simulink model "OPSPACE_Control"  (R2022b)
settings: Solver=VariableStepAuto  StartTime=0.0  StopTime=70  RelTol=1e-3
values from neighbouring files (symbols this model uses):
  a1 = 0.5    [MODELLO_ROBOT.m]    (also in calcoloJa.m)
  a2 = 0.5    [MODELLO_ROBOT.m]    (also in calcoloJa.m)
  d0 = 1    [MODELLO_ROBOT.m]    (also in calcoloJa.m)
  Kd = diag([50 50 50 50])    [MAIN.m]
  Kp = diag([750 750 750 750])    [MAIN.m]
  q0 = [theta10; theta20; p0(3)-1; -theta10-theta20]    [MAIN.m]
undefined symbols (not defined in the file or in its folder): DiscIntNeverNeededParam
settings Model: Creator=salvatoregranata  LastModifiedBy=salvatoregranata

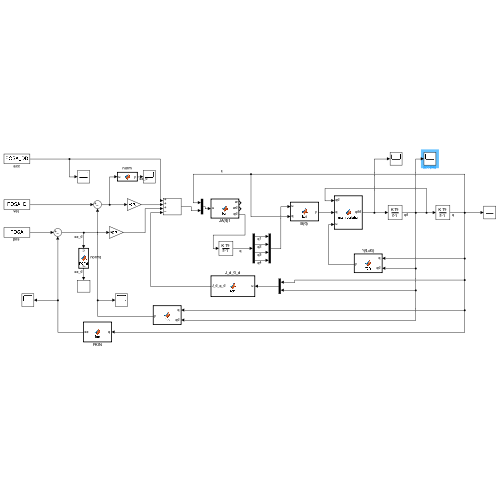
[thumbnail: Simulink's stored preview of the top-level diagram]
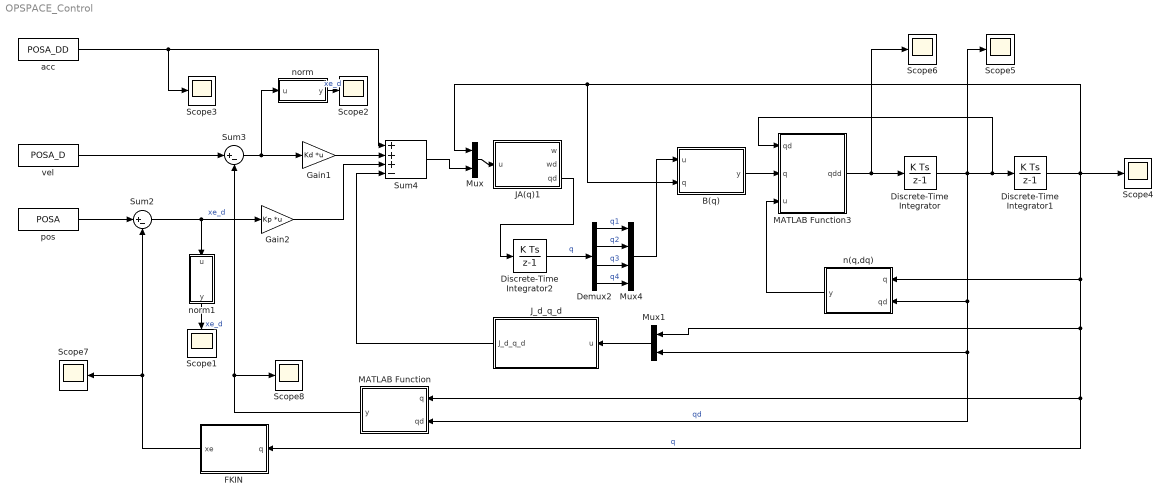
== system OPSPACE_Control ==
  B(q) : MATLAB Function  TreatAsAtomicUnit=on
  Demux2 : Demux
  Discrete-Time Integrator : DiscreteIntegrator  InitialCondition=zeros(1,4)  SampleTime=1e-3  ICPrevOutput=DiscIntNeverNeededParam  ICPrevScaledInput=DiscIntNeverNeededParam
  Discrete-Time Integrator1 : DiscreteIntegrator  InitialCondition=zeros(1,4)  SampleTime=1e-3  ICPrevOutput=DiscIntNeverNeededParam  ICPrevScaledInput=DiscIntNeverNeededParam
  Discrete-Time Integrator2 : DiscreteIntegrator  InitialCondition=q0  SampleTime=1e-3  ICPrevOutput=DiscIntNeverNeededParam  ICPrevScaledInput=DiscIntNeverNeededParam
  FKIN : MATLAB Function  TreatAsAtomicUnit=on
  Gain1 : Gain  Gain=Kd  Multiplication=Matrix(K*u)
  Gain2 : Gain  Gain=Kp  Multiplication=Matrix(K*u)
  JA(q)1 : MATLAB Function  TreatAsAtomicUnit=on
  J_d_q_d : MATLAB Function  TreatAsAtomicUnit=on
  MATLAB Function : MATLAB Function  TreatAsAtomicUnit=on
  MATLAB Function3 : MATLAB Function  TreatAsAtomicUnit=on
  Mux : Mux  Inputs=2
  Mux1 : Mux  Inputs=2
  Mux4 : Mux
  Scope{1..8} (8 alike) : Scope
  Sum2 : Sum  Inputs=|+-
  Sum3 : Sum  Inputs=|+-
  Sum4 : Sum  Inputs=+++-
  acc : FromWorkspace  VariableName=POSA_DD  SampleTime=0.001
  n(q,dq) : MATLAB Function  TreatAsAtomicUnit=on
  norm : MATLAB Function  TreatAsAtomicUnit=on
  norm1 : MATLAB Function  TreatAsAtomicUnit=on
  "pos " : FromWorkspace  VariableName=POSA  SampleTime=0.001
  "vel " : FromWorkspace  VariableName=POSA_D  SampleTime=0.001
  wires:
  acc/1 -> Scope3/1, Sum4/1
  Gain2/1 -> Sum4/3
  "pos "/1 -> Sum2/1
  Gain1/1 -> Sum4/2
  Sum3/1 -> Gain1/1, norm/1(u)
  "vel "/1 -> Sum3/1
  J_d_q_d/1(J_d_q_d) -> Sum4/4
  FKIN/1(xe) -> Scope7/1, Sum2/2
  B(q)/1(y) -> MATLAB Function3/2(q)
  MATLAB Function3/1(qdd) -> Scope6/1, Discrete-Time Integrator/1
  Discrete-Time Integrator/1 -> MATLAB Function/2(qd), Mux1/2, n(q,dq)/2(qd), Scope5/1, MATLAB Function3/1(qd), Discrete-Time Integrator1/1  "qd"
  n(q,dq)/1(y) -> MATLAB Function3/3(u)
  Discrete-Time Integrator1/1 -> Mux/1, B(q)/2(q), Scope4/1, Mux1/1, MATLAB Function/1(q), FKIN/1(q), n(q,dq)/1(q)  "q"
  MATLAB Function/1(y) -> Scope8/1, Sum3/2
  Mux/1 -> JA(q)1/1(u)
  Sum4/1 -> Mux/2
  Mux1/1 -> J_d_q_d/1(u)
  JA(q)1/3(qd) -> Discrete-Time Integrator2/1
  Demux2/1 -> Mux4/1  "q1"
  Demux2/3 -> Mux4/3  "q3"
  Demux2/4 -> Mux4/4  "q4"
  Discrete-Time Integrator2/1 -> Demux2/1  "q"
  Demux2/2 -> Mux4/2  "q2"
  Mux4/1 -> B(q)/1(u)
  norm/1(y) -> Scope2/1  "xe_d"
  Sum2/1 -> norm1/1(u), Gain2/1  "xe_d"
  norm1/1(y) -> Scope1/1  "xe_d"

== matlab function OPSPACE_Control/J_d_q_d ==
  data: u input; J_d_q_d output
function J_d_q_d = fcn(u)
a1=0.5;
a2=0.5;
q = u(1:4);
q1_d=u(5);
q2_d=u(6);
u2 = u(5:8);
% Jacobiano derivato
               
J_d = [ (-q1_d + q2_d)*(a2*cos(q(1)+q(2)))-q1_d*a1*cos(q(1)),  -(q1_d+q2_d)*(a2*cos(q(1)+q(2))),   0,  0;
         -(q1_d+q2_d)*(a2*sin(q(1)+q(2)))-q1_d*a1*sin(q(1)),  -(q1_d+q2_d)*(a2*sin(q(1)+q(2))),   0,  0;
         0, 0, 0, 0;
         0, 0, 0, 0;];
               
J_d_q_d = J_d*u2;
    
end

== matlab function OPSPACE_Control/FKIN ==
  data: q input; xe output; a2 parameter; a1 parameter; d0 parameter
function xe = fcn(q, a2, a1, d0)

theta1 = q(1);
theta2 = q(2);
d3 = q(3);
theta4 = q(4);

% Cinematica diretta
xe = [a1*cos(theta1)+a2*cos(theta1+theta2) ;
      a1*sin(theta1)+a2*sin(theta1+theta2) ;
      d3+d0;
      theta1+theta2+theta4; ];
end

== matlab function OPSPACE_Control/B(q) ==
  data: u input; y output; q input
function y = fcn(u,q)

q_1=q(1);
q_2=q(2);
q_3=q(3);
q_4=q(4);

%B è ottenuta da subs(B,pigreco,param_esatti)
B=[(45*cos(q_2))/4 + 25421/1000, (45*cos(q_2))/8 + 20177/2000,  1/4, 51/50;
(45*cos(q_2))/8 + 20177/2000,                   20177/2000,  1/4, 51/50;
                         1/4,                          1/4, 45/2,     0;
                       51/50,                        51/50,    0,   7/5]; 

y=B*u;

== matlab function OPSPACE_Control/MATLAB Function3 ==
  data: qd input; q input; u input; qdd output
function qdd = manipulator(qd, q, u)

q_1 = q(1);
q_2 = q(2);
q_3 = q(3);
q_4 = q(4);
qd_1 = qd(1);
qd_2 = qd(2);
qd_3 = qd(3);
qd_4 = qd(4);

   
n = [ qd_1/10000 - (51*qd_1*qd_2*sin(q_2))/8 - (qd_2*sin(q_2)*(51*qd_1 + 51*qd_2))/8;
                                                 (51*sin(q_2)*qd_1^2)/8 + qd_2/10000;
                                                                  4*qd_3 + 12753/100;
                                                                              2*qd_4];
 
                                                                    
B = [ (51*cos(q_2))/4 + 26921/1000, (51*cos(q_2))/8 + 21677/2000,  1/4, 51/50;
      (51*cos(q_2))/8 + 21677/2000,                   21677/2000,  1/4, 51/50;
                               1/4,                          1/4, 51/2,     0;
                             51/50,                        51/50,    0,   7/5];
 
qdd = inv(B)*(u-n);

== matlab function OPSPACE_Control/n(q,dq) ==
  data: q input; y output; qd input
function y = fcn(q,qd)
qd_1 = qd(1);
qd_2 = qd(2);
qd_3 = qd(3);
qd_4 = qd(4);
q_1 = q(1);
q_2 = q(2);
q_3 = q(3);
q_4 = q(4);
   
n = [ qd_1/10000 - (51*qd_1*qd_2*sin(q_2))/8 - (qd_2*sin(q_2)*(51*qd_1 + 51*qd_2))/8;
                                                 (51*sin(q_2)*qd_1^2)/8 + qd_2/10000;
                                                                  4*qd_3 + 12753/100;
                                                                              2*qd_4];
y = n;

== matlab function OPSPACE_Control/MATLAB Function ==
  data: q input; qd input; y output
function y = fcn(q,qd)

theta1=q(1);
theta2=q(2);
d3=q(3);
theta4=q(4);

k=1;

d0=1;
a1=0.5;
a2=a1;

%calcolo le matrici di trasformazione tra i frame dei giunti
A01=[cos(theta1) -sin(theta1) 0 a1*cos(theta1); sin(theta1) cos(theta1) 0 a1*sin(theta1); 0 0 1 0; 0 0 0 1];
A12=[cos(theta2) sin(theta2) 0 a2*cos(theta2); sin(theta2) -cos(theta2) 0 a2*sin(theta2); 0 0 -1 0; 0 0 0 1];
A23=[1 0 0 0; 0 1 0 0; 0 0 1 d3; 0 0 0 1];
A34=[cos(theta4) -sin(theta4) 0 0; sin(theta4) cos(theta4) 0 0; 0 0 1 0; 0 0 0 1];

AB0=[1 0 0 0; 0 1 0 0; 0 0 1 d0; 0 0 0 1];

A02=A01*A12;
A03=A02*A23;
A04=A03*A34;

AB1=AB0*A01;
AB2=AB0*A02;
AB3=AB0*A03;
AB4=AB0*A04;

%calcolo i vettori posizione dei frame rispetto al frame 0
pB0=[0;0;d0];

p1=A01(1:3,4);
p2=A02(1:3,4);
p3=A03(1:3,4);
p4=A04(1:3,4);

pB1=AB1(1:3,4);
pB2=AB2(1:3,4);
pB3=AB3(1:3,4);
pB4=AB4(1:3,4);


%===calcolo dello Jacobiano===

%versori z:
z0=[0;0;1];
z1=z0;
z2=-z1;
z3=z2;

%componenti lineari dello jacobiano
JP1=cross(z0,p4-pB0);
JP2=cross(z1,p4-p1);
JP3=z2;
JP4=cross(z3,p4-p3);

%componenti angolari dello jacobiano

JO1=z0; 
JO2=z1;
JO3=[0;0;0];
JO4=z3;

J=[JP1 JP2 JP3 JP4; JO1 JO2 JO3 JO4];
Jridotta=[J(1:3,:);J(6,:)];

y = Jridotta*qd;

== matlab function OPSPACE_Control/JA(q)1 ==
  data: u input; w output; wd output; qd output
function [w,wd, qd] = fcn(u)
q = u(1:4);
u2 = u(5:8);

d0 = 1;
d1 = 0;
d2 = 0;
d3 = 0;
d4 = 0;

alpha1 = 0;
alpha2 = pi;
alpha3 = 0;
alpha4 = 0;

a1 = 0.5;
a2 = 0.5;
a3 = 0;
a4 = 0;

% Jacobiano
J = [ -a1*sin(q(1))-a2*sin(q(1)+q(2))   -a2*sin(q(1)+q(2))  0   0   ;
       a1*cos(q(1))+a2*cos(q(1)+q(2))    a2*cos(q(1)+q(2))  0   0   ;
                   0                              0         1   0   ;
                   1                              1         0   1   ];
w=abs(det(J));              
wd = [0; a1*a2*cos(q(2)); 0; 0];
               
% Damped Least Squares
intervallo = 0.001;
k = 0.1;

if(abs(det(J))) < intervallo
    J = J' * inv(J*J' + eye(4)*k^2);
    qd = J*(u2);
else
    qd = inv(J)*(u2);
end
y = u;

== matlab function OPSPACE_Control/norm ==
  data: u input; y output
function y = norm(u)
y = norm(u);

== matlab function OPSPACE_Control/norm1 ==
  data: u input; y output
function y = norm(u)
y = norm(u);
